simulink model "sfun_storageTnodes_AW"  (R2013b)
settings: Solver=ode45  StartTime=0.0  StopTime=10.0  RelTol=1e-3
settings Model: Creator=awohlfei  LastModifiedBy=drhf
settings DebuggingCC: StateNameClashWarn=warning

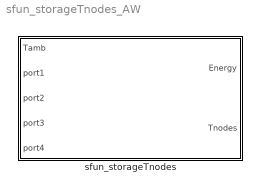
== system sfun_storageTnodes_AW ==
  sfun_storageTnodes : Subsystem  mask{dia=0.5, volume=0.5, standing=1, uloss=100, ubot=100, utop=100, cond=0.63, tini=20, nodes=100, nconnect=4}
      mask prompts: dia "diameter [m]"; volume "volume [m³]"; standing "standing cylinder"; uloss "heat transfer coefficient to ambient [W/m²K]"; ubot "heat transfer coefficient to ambient bottom [W/m²K]"; utop "heat transfer coefficient to ambient top [W/m²K]"; cond "effective thermal conductivity [W/mK]"; tini "initial temperature [°C]"; nodes "number of nodes [1]"; nconnect "number of ports [1]"
      mask init:
      | if (floor(nodes)-nodes>eps(nodes)) || nodes < 1.0
      |     error('The number of nodes must be a positve integer!');
      | end
      | 
      | if (floor(nconnect)-nconnect>eps(nconnect)) || nconnect < 1.0
      |     error('The number of ports must be a positve integer!');
      | end
      | 
      | 
      | 
      | if numel(tini)==1
      |     tini = ones(int32(nodes), 1)*tini;
      | else
      |     if numel(tini)~=int32(nodes)
      |         error('The initialisation temperature must be a scalar or a vector of size of number of nodes!');
      |     end
      | end
      | 
      | CarnotCallbacks_storage_Tnodes('InitCallback', gcb, nconnect);

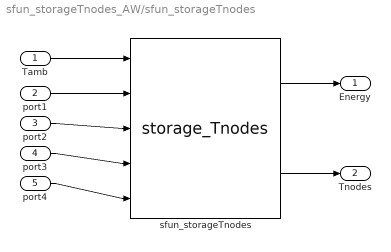
== system sfun_storageTnodes_AW/sfun_storageTnodes ==
  Tamb : Inport
  port1 : Inport  Port=2
  port2 : Inport  Port=3
  port3 : Inport  Port=4
  port4 : Inport  Port=5
  sfun_storageTnodes : S-Function  FunctionName=storage_Tnodes  Parameters=dia, volume, standing, uloss , ubot, utop, cond, tini, nodes, nconnect  EnableBusSupport=off
  Energy : Outport
  Tnodes : Outport  Port=2
  wires:
  sfun_storageTnodes/1 -> Energy/1
  sfun_storageTnodes/2 -> Tnodes/1
  Tamb/1 -> sfun_storageTnodes/1
  port1/1 -> sfun_storageTnodes/2
  port2/1 -> sfun_storageTnodes/3
  port3/1 -> sfun_storageTnodes/4
  port4/1 -> sfun_storageTnodes/5
